simulink model "igbtforrload"  (R2016a)
settings: Solver=VariableStepAuto  StartTime=0.0  StopTime=10.0  RelTol=1e-3
libraries: powerlib x9, simulink x3
settings Model: Creator=Admin  LastModifiedBy=ADITYA

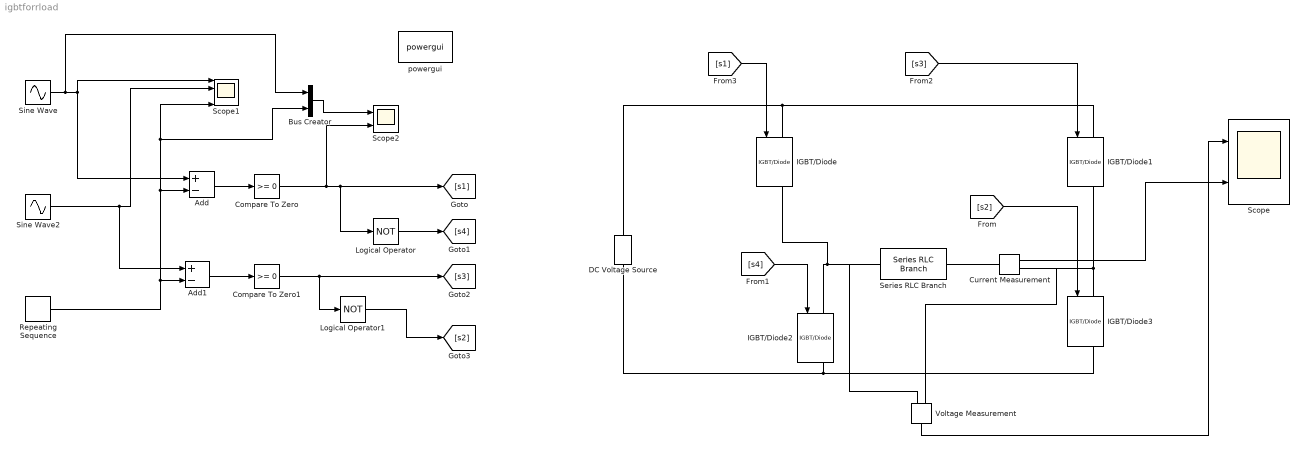
== system igbtforrload ==
  Add : Sum  Inputs=+-
  Add1 : Sum  Inputs=+-
  Bus Creator : BusCreator  Inputs=2
  Compare To Zero : simulink/Logic and Bit Operations/Compare To Zero  relop=>=  OutDataTypeStr=boolean
  Compare To Zero1 : simulink/Logic and Bit Operations/Compare To Zero  relop=>=  OutDataTypeStr=boolean
  Current Measurement : powerlib/Measurements/Current Measurement  PhasorSimulation=off  OutputType=Complex  PSBequivalent=0
  DC Voltage Source : powerlib/Electrical Sources/DC Voltage Source  Amplitude=400  Measurements=None
  IGBT/Diode{,1..3} (4 alike) : powerlib/Power Electronics/IGBT//Diode  Ron=1e-3  Rs=1e5  Cs=inf  Measurements=on
  Logical Operator : Logic  Operator=NOT  AllPortsSameDT=off  OutDataTypeStr=boolean
  Logical Operator1 : Logic  Operator=NOT  AllPortsSameDT=off  OutDataTypeStr=boolean
  Repeating Sequence : simulink/Sources/Repeating Sequence  rep_seq_t=[0 2]  rep_seq_y=[0 2]
  Scope : Scope  NumInputPorts=2
  Scope1 : Scope  NumInputPorts=4
  Scope2 : Scope  NumInputPorts=2
  Series RLC Branch : powerlib/Elements/Series RLC Branch  LConnTagsString=__new0  RConnTagsString=__new0  BranchType=R  Resistance=5  Inductance=1e-3  SetiL0=off  InitialCurrent=0  Capacitance=1e-6  Setx0=off  InitialVoltage=0  Measurements=Branch voltage and current
  Sine Wave : Sin  Amplitude=100  Phase=150  SampleTime=0.01
  Sine Wave2 : Sin  SineType=Sample based  Amplitude=100  Phase=60  Samples=150  SampleTime=0.01
  Voltage Measurement : powerlib/Measurements/Voltage Measurement  PhasorSimulation=off  OutputType=Complex  PSBequivalent=0
  powergui : powerlib/powergui  Priority=1  SimulationMode=Continuous  SolverType=Tustin/Backward Euler (TBE)  SampleTime=50e-6  frequency=60  SPID=off  DisableSnubberDevices=off  DisableRonSwitches=off  DisableVfSwitches=off  SwTol=0  DisplayEquations=off  Interpol=off  ExternalGateDelay=off  methode=off  Ts=10  FunctionMessages=off  echomessages=off  HookPort=off  EnableUseOfTLC=off  x0status=blocks  frequencyindice=0  Pbase=100e6  ErrMax=1e-4  Iterations=50  UnitsV=kV  UnitsW=MW  buscounter=0  RestoreLinks=warning  ResistiveCurrentMeasurement=off  Frange=[0:2:500]  Ylog=off  Xlog=on  ShowGrid=off  save=off  variable=ZData  structure=0  ZoomFFT=off  StartTime=0.0  cycles=1  DisplayStyle=1  fundamental=60  FreqAxis=off  MaxFrequency=1000  frequencyindicesteady=1  RmsSteady=1  display=off
  wires:
  [s1] -> IGBT/Diode/1
  [s3] -> IGBT/Diode1/1
  [s4] -> IGBT/Diode2/1
  [s2] -> IGBT/Diode3/1
  Voltage Measurement/1 -> Scope/1
  Current Measurement/1 -> Scope/2
  Sine Wave/1 -> Bus Creator/1, Add/1, Scope1/1
  Sine Wave2/1 -> Add1/1, Scope1/2
  Add/1 -> Compare To Zero/1
  Add1/1 -> Compare To Zero1/1
  Logical Operator/1 -> [s4]
  Compare To Zero1/1 -> Logical Operator1/1, [s3]
  Logical Operator1/1 -> [s2]
  Compare To Zero/1 -> Scope2/2, Logical Operator/1, [s1]
  Bus Creator/1 -> Scope2/1
  Repeating Sequence/1 -> Add1/2, Add/2, Bus Creator/2, Scope1/4
  connections:
  DC Voltage Source/RConn1 -- IGBT/Diode1/LConn1 -- IGBT/Diode/LConn1
  IGBT/Diode/RConn1 -- Voltage Measurement/LConn2 -- Series RLC Branch/LConn1 -- IGBT/Diode2/LConn1
  Current Measurement/LConn1 -- Series RLC Branch/RConn1
  IGBT/Diode1/RConn1 -- Current Measurement/RConn1 -- Voltage Measurement/LConn1 -- IGBT/Diode3/LConn1
  DC Voltage Source/LConn1 -- IGBT/Diode2/RConn1 -- IGBT/Diode3/RConn1
